simulink model "Ecuacion_Ejercicio_1"  (R2017b)
settings: Solver=VariableStepAuto  StartTime=0.0  StopTime=10.0  RelTol=1e-3
settings Model: Creator=Elmer  LastModifiedBy=Elmer

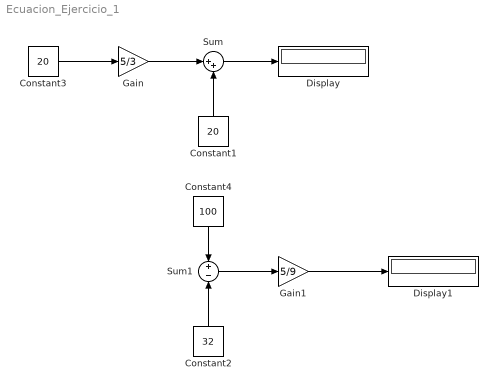
== system Ecuacion_Ejercicio_1 ==
  Constant1 : Constant  Value=20
  Constant2 : Constant  Value=32
  Constant3 : Constant  Value=20
  Constant4 : Constant  Value=100
  Display : Display
  Display1 : Display
  Gain : Gain  Gain=5/3
  Gain1 : Gain  Gain=5/9
  Sum : Sum  Inputs=|++
  Sum1 : Sum  Inputs=+-
  wires:
  Constant3/1 -> Gain/1
  Gain/1 -> Sum/1
  Constant1/1 -> Sum/2
  Sum/1 -> Display/1
  Gain1/1 -> Display1/1
  Constant2/1 -> Sum1/2
  Sum1/1 -> Gain1/1
  Constant4/1 -> Sum1/1
